simulink model "BLDC_equ"  (R2023a)
settings: Solver=VariableStepAuto  StartTime=0.0  StopTime=10  RelTol=1e-6
undefined symbols (not defined in the file): J_rot, K_m, R_3ph, T_q
settings Model: Creator=Artem Sannikov  LastModifiedBy=Artem Sannikov

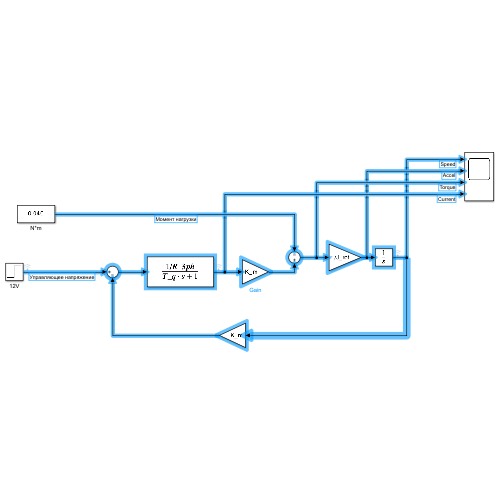
[thumbnail: Simulink's stored preview of the top-level diagram]
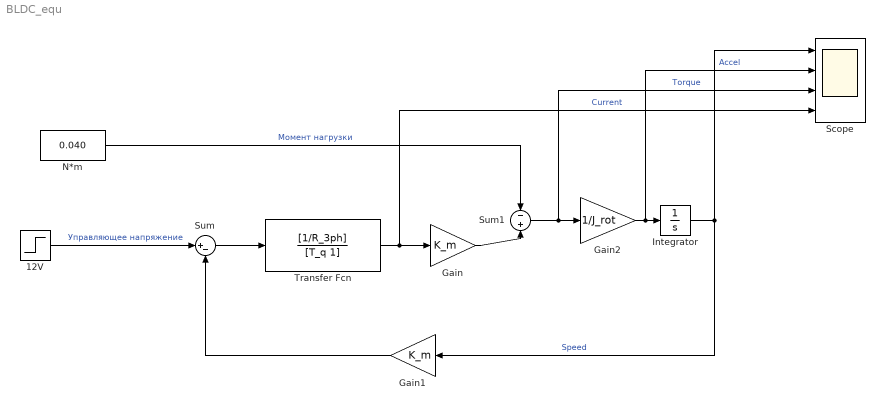
== system BLDC_equ ==
  12V : Step  After=12  SampleTime=0
  Gain : Gain  Gain=K_m
  Gain1 : Gain  Gain=K_m
  Gain2 : Gain  Gain=1/J_rot
  Integrator : Integrator
  N*m : Constant  Value=0.040
  Scope : Scope  NumInputPorts=4
  Sum : Sum  Inputs=|+-
  Sum1 : Sum  Inputs=-|+
  Transfer Fcn : TransferFcn  Numerator=[1/R_3ph]  Denominator=[T_q 1]
  wires:
  Integrator/1 -> Scope/1, Gain1/1  "Speed"
  Gain2/1 -> Scope/2, Integrator/1  "Accel"
  Sum1/1 -> Scope/3, Gain2/1  "Torque"
  Transfer Fcn/1 -> Scope/4, Gain/1  "Current"
  Gain1/1 -> Sum/2
  12V/1 -> Sum/1  "Управляющее напряжение"
  N*m/1 -> Sum1/1  "Момент нагрузки"
  Sum/1 -> Transfer Fcn/1
  Gain/1 -> Sum1/2
